simulink model "az_INDI_controller"  (R2023b)
settings: Solver=FixedStepAuto  StartTime=0.0  StopTime=8  FixedStep=0.001  RelTol=1e-3  AbsTol=1e-6
PreLoadFcn:
  | %aero_guid_dat
StopFcn:
  | %aero_guid_plot
undefined symbols (not defined in the file or in its folder): alpha_vec, Cm_alpha, Cm_el, Cm_q, Cx_alpha, Cz_alpha, Cz_el, d_ref, fin_max, fin_maxrate, fin_min, g, h_ini, Iyy, l_acc, Mach_vec, mass, q_ini, S_ref, Thrust, v_ini, x_ini
libraries: aerolibasang x3, aerolibatmos2 x1, aerolibactuator x1, simulink x1
CloseFcn:
  | h=findobj('type','figure');if ~isempty(h);close(h);end
Description:
  | Dynamics of a missile engaging a target which is flying straight and level
settings Model: Creator=The MathWorks, Inc.  LastModifiedBy=luzhi
settings SolverCC: AutoScaleAbsTol=off  AlgebraicLoopSolver=TrustRegion
settings DataIOCC: SaveFormat=Array  SaveOutput=off  ReturnWorkspaceOutputs=off  StateSaveName=xbase  OutputSaveName=ybase  SignalLoggingName=sigsOut
settings OptimizationCC: BlockReduction=off  ReuseModelBlockBuffer=off  ExpressionDepthLimit=2147483647  InitFltsAndDblsToZero=on  LifeSpan=inf
settings DebuggingCC: SaveWithParameterizedLinksMsg=none  SignalResolutionControl=TryResolveAllWithWarning  MultiTaskDSMMsg=warning  MultiTaskCondExecSysMsg=none  SigSpecEnsureSampleTimeMsg=none  FcnCallInpInsideContextMsg=warning  UnconnectedInputMsg=warning  UnconnectedOutputMsg=warning  UnconnectedLineMsg=warning  StateNameClashWarn=warning  SFUnexpectedBacktrackingDiag=warning  SFNoUnconditionalDefaultTransitionDiag=warning  SFExecutionAtInitializationDiag=none  ArithmeticOperatorsInVariantConditions=warning
settings HardwareCC: ProdBitPerPointer=32  ProdBitPerSizeT=32  ProdBitPerPtrDiffT=32  ProdLargestAtomicFloat=None  ProdIntDivRoundTo=Undefined  ProdEndianess=Unspecified  ProdWordSize=32  ProdHWDeviceType=32-bit Generic
settings ModelReferenceCC: EnableRefExpFcnMdlSchedulingChecks=on  PropagateSignalLabelsOutOfModel=off
settings SFSimCC: SimUseLocalCustomCode=off  SimParseCustomCode=off  CustomCodeUndefinedFunction=UseInterfaceOnly
settings RTWCC: RTWUseLocalCustomCode=off
settings CodeAppCC: StateflowObjectComments=on
settings GRTTargetCC: TargetFcnLib=ansi_tfl_tmw.mat  TargetLangStandard=C89/C90 (ANSI)  CombineOutputUpdateFcns=off  GRTInterface=on
settings ConfigComp: CovMetricSettings=d  CovSaveCumulativeToWorkspaceVar=on  CovSaveSingleToWorkspaceVar=on  CovExternalEMLEnable=off  CovSFcnEnable=off

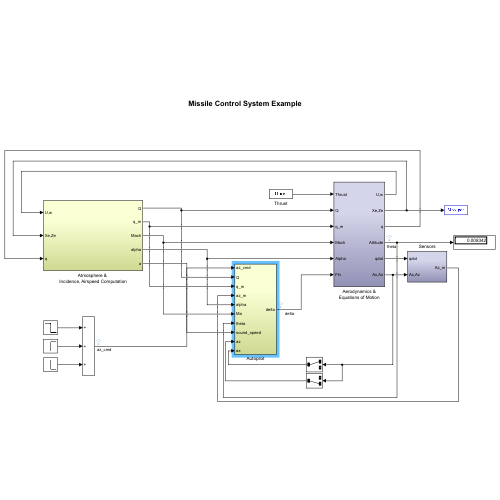
[thumbnail: Simulink's stored preview of the top-level diagram]
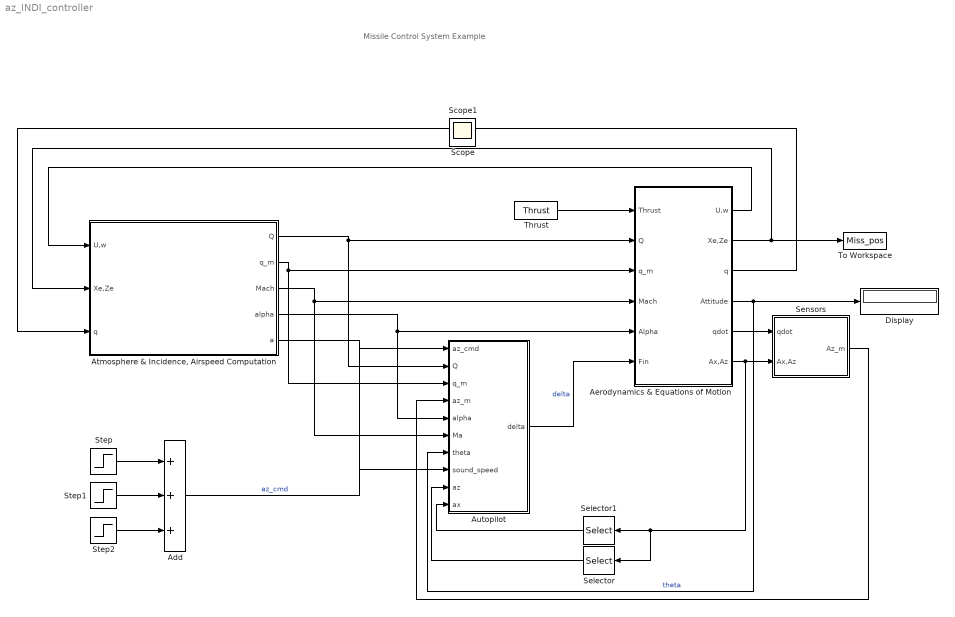
== system az_INDI_controller ==
  note: Missile Control System Example
  Add : Sum  Inputs=3
  Aerodynamics & Equations of Motion : Subsystem
  "Atmosphere & Incidence, Airspeed Computation" : Subsystem
  Autopilot : Subsystem
  Display : Display
  Selector : Selector  InputPortWidth=2  IndexOptions=Index vector (dialog)  Indices=[2]  OutputSizes=1
  Selector1 : Selector  InputPortWidth=2  IndexOptions=Index vector (dialog)  Indices=1  OutputSizes=1
  Sensors : Subsystem
  Step : Step  After=-10  SampleTime=0
  Step1 : Step  Time=3  After=20  SampleTime=0
  Step2 : Step  Time=5  After=-10  SampleTime=0
  Thrust : Constant  Value=Thrust
  To Workspace : ToWorkspace  VariableName=Miss_pos  SaveFormat=Structure With Time  SampleTime=-1
  Scope : Scope
  Scope1 : Scope
  wires:
  Autopilot/1(delta) -> Aerodynamics & Equations of Motion/6(Fin)  "delta"
  Aerodynamics & Equations of Motion/6(Ax,Az) -> Selector1/1, Selector/1, Sensors/2(Ax,Az)
  Aerodynamics & Equations of Motion/5(qdot) -> Sensors/1(qdot)
  Aerodynamics & Equations of Motion/4(Attitude) -> Autopilot/7(theta), Display/1  "theta"
  "Atmosphere & Incidence, Airspeed Computation"/2(q_m) -> Aerodynamics & Equations of Motion/3(q_m), Autopilot/3(q_m)
  "Atmosphere & Incidence, Airspeed Computation"/4(alpha) -> Autopilot/5(alpha), Aerodynamics & Equations of Motion/5(Alpha)
  "Atmosphere & Incidence, Airspeed Computation"/1(Q) -> Autopilot/2(Q), Aerodynamics & Equations of Motion/2(Q)
  Aerodynamics & Equations of Motion/1(U,w) -> "Atmosphere & Incidence, Airspeed Computation"/1(U,w)
  "Atmosphere & Incidence, Airspeed Computation"/3(Mach) -> Autopilot/6(Ma), Aerodynamics & Equations of Motion/4(Mach)
  Aerodynamics & Equations of Motion/2(Xe,Ze) -> To Workspace/1, "Atmosphere & Incidence, Airspeed Computation"/2(Xe,Ze)
  Aerodynamics & Equations of Motion/3(q) -> "Atmosphere & Incidence, Airspeed Computation"/3(q)
  Thrust/1 -> Aerodynamics & Equations of Motion/1(Thrust)
  Sensors/1(Az_m) -> Autopilot/4(az_m)
  "Atmosphere & Incidence, Airspeed Computation"/5(a) -> Autopilot/8(sound_speed)
  Selector/1 -> Autopilot/9(az)
  Add/1 -> Autopilot/1(az_cmd)  "az_cmd"
  Step/1 -> Add/1
  Step1/1 -> Add/2
  Step2/1 -> Add/3
  Selector1/1 -> Autopilot/10(ax)

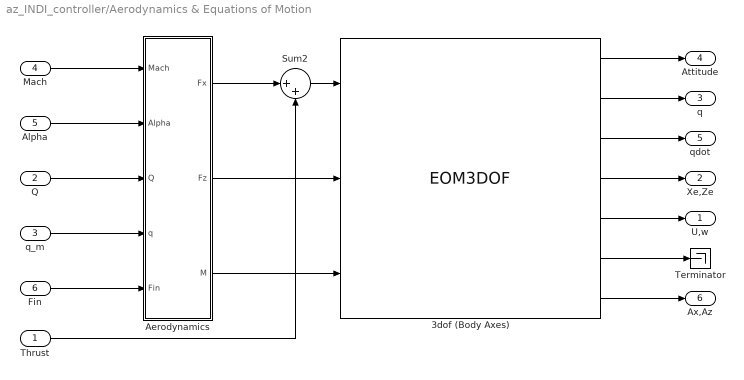
== system az_INDI_controller/Aerodynamics & Equations of Motion ==
  Thrust : Inport
  Q : Inport  Port=2
  q_m : Inport  Port=3
  Mach : Inport  Port=4
  Alpha : Inport  Port=5
  Fin : Inport  Port=6
  3dof (Body Axes) : EOM3DOF  v_ini=v_ini  theta_ini=theta_ini  q_ini=q_ini  alpha_ini=alpha_ini  pos_ini=[x_ini -h_ini]  mass=mass  Iyy=Iyy  g=g  abi_flag=on
  Aerodynamics : Subsystem
  Sum2 : Sum  Inputs=|++  InputSameDT=on  SaturateOnIntegerOverflow=on  OutDataTypeStr=Inherit: Same as first input
  Terminator : Terminator
  U,w : Outport  InitialOutput=0  VectorParamsAs1DForOutWhenUnconnected=off
  Xe,Ze : Outport  Port=2  InitialOutput=0  VectorParamsAs1DForOutWhenUnconnected=off
  q : Outport  Port=3  InitialOutput=0  VectorParamsAs1DForOutWhenUnconnected=off
  Attitude : Outport  Port=4  InitialOutput=0  VectorParamsAs1DForOutWhenUnconnected=off
  qdot : Outport  Port=5  InitialOutput=0  VectorParamsAs1DForOutWhenUnconnected=off
  Ax,Az : Outport  Port=6  InitialOutput=0  VectorParamsAs1DForOutWhenUnconnected=off
  wires:
  Aerodynamics/3(" M") -> 3dof (Body Axes)/3
  Sum2/1 -> 3dof (Body Axes)/1
  Fin/1 -> Aerodynamics/5(Fin)
  Aerodynamics/2(Fz) -> 3dof (Body Axes)/2
  Aerodynamics/1(Fx) -> Sum2/1
  Thrust/1 -> Sum2/2
  q_m/1 -> Aerodynamics/4(q)
  Mach/1 -> Aerodynamics/1(Mach)
  Q/1 -> Aerodynamics/3(Q)
  Alpha/1 -> Aerodynamics/2(Alpha)
  3dof (Body Axes)/7 -> Ax,Az/1
  3dof (Body Axes)/6 -> Terminator/1
  3dof (Body Axes)/5 -> U,w/1
  3dof (Body Axes)/4 -> Xe,Ze/1
  3dof (Body Axes)/3 -> qdot/1
  3dof (Body Axes)/2 -> q/1
  3dof (Body Axes)/1 -> Attitude/1

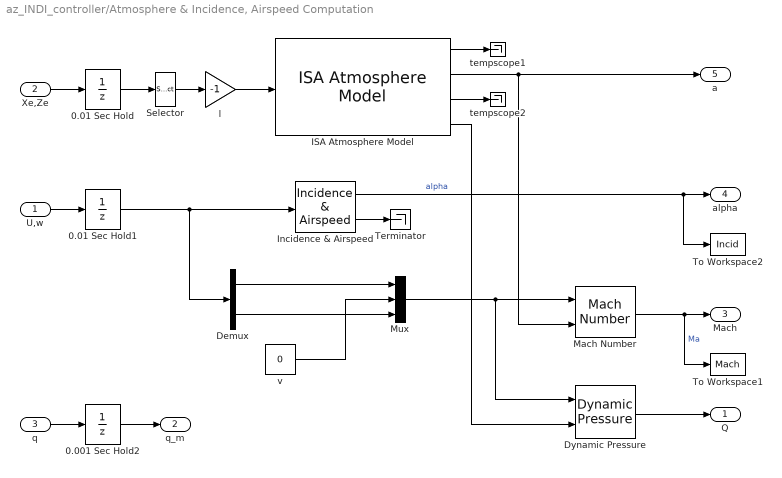
== system az_INDI_controller/Atmosphere & Incidence, Airspeed Computation ==
  U,w : Inport
  Xe,Ze : Inport  Port=2
  q : Inport  Port=3
  0.001 Sec Hold2 : UnitDelay  InitialCondition=q_ini  SampleTime=0.001  HasFrameUpgradeWarning=on
  0.01 Sec Hold : UnitDelay  InitialCondition=[x_ini -h_ini]  SampleTime=0.01  HasFrameUpgradeWarning=on
  0.01 Sec Hold1 : UnitDelay  InitialCondition=[v_ini 0]  SampleTime=0.01  HasFrameUpgradeWarning=on
  Demux : Demux  Outputs=2
  Dynamic Pressure : aerolibasang/Dynamic Pressure
  ISA Atmosphere Model : aerolibatmos2/ISA Atmosphere Model  useExtended=off  action=Warning  custom=off  viscosityOut=off  g=9.80665  gamma=1.4  R=287.0531  L=0.0065  h_trop=11000  h_strat=20000  rho0=1.225  P0=101325  T0=288.15  h0=0
  Incidence & Airspeed : aerolibasang/Incidence  & Airspeed
  Mach Number : aerolibasang/Mach Number
  Mux : Mux  Inputs=3
  Selector : Selector  InputPortWidth=2  IndexOptions=Index vector (dialog)  Indices=[2]  OutputSizes=1
  Terminator : Terminator
  To Workspace1 : ToWorkspace  VariableName=Mach  SaveFormat=Structure With Time  SampleTime=-1
  To Workspace2 : ToWorkspace  VariableName=Incid  SaveFormat=Structure With Time  SampleTime=-1
  l : Gain  Gain=-1  SaturateOnIntegerOverflow=on  OutDataTypeStr=Inherit: Same as input  ParamDataTypeStr=Inherit: Same as input
  tempscope1 : Terminator
  tempscope2 : Terminator
  v : Constant  Value=0
  Q : Outport
  q_m : Outport  Port=2
  Mach : Outport  Port=3
  alpha : Outport  Port=4
  a : Outport  Port=5
  wires:
  U,w/1 -> 0.01 Sec Hold1/1
  Incidence & Airspeed/1 -> To Workspace2/1, alpha/1  "alpha"
  Demux/1 -> Mux/1
  Demux/2 -> Mux/3
  v/1 -> Mux/2
  Mux/1 -> Mach Number/1, Dynamic Pressure/1
  Incidence & Airspeed/2 -> Terminator/1
  ISA Atmosphere Model/4 -> Dynamic Pressure/2
  Mach Number/1 -> To Workspace1/1, Mach/1  "Ma"
  Dynamic Pressure/1 -> Q/1
  0.01 Sec Hold1/1 -> Incidence & Airspeed/1, Demux/1
  0.01 Sec Hold/1 -> Selector/1
  l/1 -> ISA Atmosphere Model/1
  ISA Atmosphere Model/1 -> tempscope1/1
  ISA Atmosphere Model/3 -> tempscope2/1
  Selector/1 -> l/1
  Xe,Ze/1 -> 0.01 Sec Hold/1
  ISA Atmosphere Model/2 -> a/1, Mach Number/2
  0.001 Sec Hold2/1 -> q_m/1
  q/1 -> 0.001 Sec Hold2/1

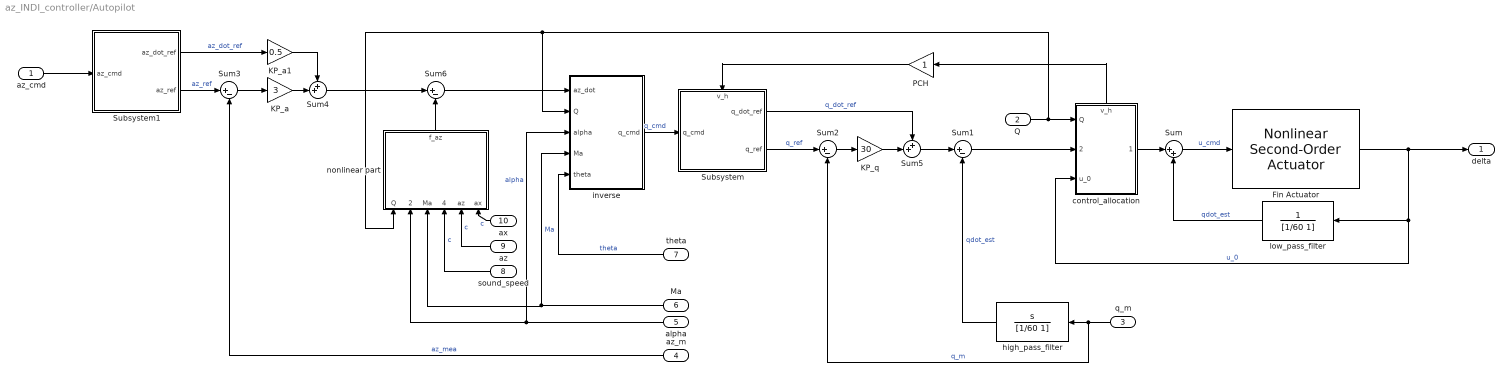
== system az_INDI_controller/Autopilot ==
  az_cmd : Inport
  Q : Inport  Port=2
  q_m : Inport  Port=3
  az_m : Inport  Port=4
  alpha : Inport  Port=5
  Ma : Inport  Port=6
  theta : Inport  Port=7
  sound_speed : Inport  Port=8
  az : Inport  Port=9
  ax : Inport  Port=10
  Fin Actuator : aerolibactuator/Nonlinear Second-Order Actuator  wn_fin=wn_fin  z_fin=z_fin  fin_max=fin_max  fin_min=fin_min  fin_maxrate=fin_maxrate  fin_act_0=fin_act_0  fin_act_vel=0
  KP_a : Gain  Gain=3
  KP_a1 : Gain  Gain=0.5
  KP_q : Gain  Gain=30
  PCH : Gain
  Subsystem : Subsystem
      settings: PortSchema="{\"entries\":[{\"content\":{\"sides\":[{\"content\":{\"connectorIds\":[\"In1\"]},\"type\":\"ConnectorPlacement.EquallySpacedRectSide\",\"uuid\":\"21326aec-3e5e-4acc-8d4b-147fb67c37ef\"},{\"content\":{\"connectorIds\":[\"Out1\",\"Out2\"],\"side\":\"RIGHT\"},\"type\":\"ConnectorPlacement.EquallySpacedRectSide\",\"uuid\":\"9c9abec6-e162-41f3-9a87-a5e646e431f6\"},{\"content\":{\"connectorIds\":[\"In2\"],\"side\":\"TOP\"},\"type\":\"ConnectorPlacement.EquallySpacedRectSide\",\"uuid\":\"37a4f4dd-e2ce-4d3c-ba5c-0e6f54d2f89b\"}]},\"type\":\"ConnectorPlacement.EquallySpacedConnector\",\"uuid\":\"006ee997-d3e3-4e6d-9e3d-0018891eb923\"}],\"packageUris\":[\"http://schema.mathworks.com/mf0/Connector/R2020b\"],\"version\":\"1.0\"}"
  Subsystem1 : Subsystem
  Sum : Sum  Inputs=|++
  Sum{1..3,6} (4 alike) : Sum  Inputs=|+-
  Sum4 : Sum  Inputs=++|
  Sum5 : Sum  Inputs=++|
  control_allocation : Subsystem
      settings: PortSchema="{\"entries\":[{\"content\":{\"sides\":[{\"content\":{\"connectorIds\":[\"In1\",\"In2\",\"In3\"]},\"type\":\"ConnectorPlacement.EquallySpacedRectSide\",\"uuid\":\"a0ce9da5-1ffc-4f75-9763-d32b58958b30\"},{\"content\":{\"connectorIds\":[\"Out1\"],\"side\":\"RIGHT\"},\"type\":\"ConnectorPlacement.EquallySpacedRectSide\",\"uuid\":\"34e52099-0fbe-4ef7-a509-693d90ad8665\"},{\"content\":{\"connectorIds\":[\"Out2\"],\"side\":\"TOP\"},\"type\":\"ConnectorPlacement.EquallySpacedRectSide\",\"uuid\":\"02b44c40-6b1e-4ed6-9dfc-88d3b20cdc66\"}]},\"type\":\"ConnectorPlacement.EquallySpacedConnector\",\"uuid\":\"9b53b305-2d8c-4631-9888-cc5118213f1a\"}],\"packageUris\":[\"http://schema.mathworks.com/mf0/Connector/R2020b\"],\"version\":\"1.0\"}"
  high_pass_filter : TransferFcn  Numerator=[1 0]  Denominator=[1/60 1]
  inverse : Subsystem
  low_pass_filter : TransferFcn  Denominator=[1/60 1]
  nonlinear part : Subsystem
  delta : Outport
  wires:
  Sum/1 -> Fin Actuator/1  "u_cmd"
  Fin Actuator/1 -> low_pass_filter/1, control_allocation/3(u_0), delta/1  "u_0"
  Q/1 -> inverse/2(Q), nonlinear part/1(Q), control_allocation/1(Q)
  Sum1/1 -> control_allocation/2(d_qdot)
  control_allocation/1(du_cmd) -> Sum/1
  high_pass_filter/1 -> Sum1/2  "qdot_est"
  q_m/1 -> Sum2/2, high_pass_filter/1  "q_m"
  low_pass_filter/1 -> Sum/2  "qdot_est"
  Sum2/1 -> KP_q/1
  KP_q/1 -> Sum5/2
  Sum5/1 -> Sum1/1
  Subsystem/1(q_dot_ref) -> Sum5/1  "q_dot_ref"
  Subsystem/2(q_ref) -> Sum2/1  "q_ref"
  control_allocation/2(v_h) -> PCH/1
  PCH/1 -> Subsystem/2(v_h)
  Subsystem1/2(az_ref) -> Sum3/1  "az_ref"
  Sum3/1 -> KP_a/1
  az_m/1 -> Sum3/2  "az_mea"
  KP_a/1 -> Sum4/2
  Subsystem1/1(az_dot_ref) -> KP_a1/1  "az_dot_ref"
  Sum4/1 -> Sum6/1
  Sum6/1 -> inverse/1(az_dot)
  inverse/1(q_cmd) -> Subsystem/1(q_cmd)  "q_cmd"
  alpha/1 -> nonlinear part/2(alpha), inverse/3(alpha)  "alpha"
  Ma/1 -> inverse/4(Ma), nonlinear part/3(Ma)  "Ma"
  theta/1 -> inverse/5(theta)  "theta"
  nonlinear part/1(f_az) -> Sum6/2
  sound_speed/1 -> nonlinear part/4(sound_speed)  "c"
  az/1 -> nonlinear part/5(az)  "c"
  ax/1 -> nonlinear part/6(ax)  "c"
  KP_a1/1 -> Sum4/1
  az_cmd/1 -> Subsystem1/1(az_cmd)

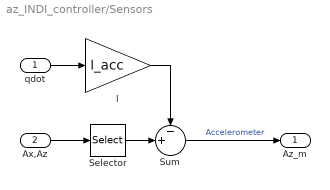
== system az_INDI_controller/Sensors ==
  qdot : Inport
  Ax,Az : Inport  Port=2
  Selector : Selector  InputPortWidth=2  IndexOptions=Index vector (dialog)  Indices=[2]  OutputSizes=1
  Sum : Sum  Inputs=-+|  InputSameDT=on  SaturateOnIntegerOverflow=on  OutDataTypeStr=Inherit: Same as first input
  l : Gain  Gain=l_acc  SaturateOnIntegerOverflow=on  OutDataTypeStr=Inherit: Same as input  ParamDataTypeStr=Inherit: Same as input
  Az_m : Outport  InitialOutput=0  VectorParamsAs1DForOutWhenUnconnected=off
  wires:
  Selector/1 -> Sum/2
  Ax,Az/1 -> Selector/1
  l/1 -> Sum/1
  Sum/1 -> Az_m/1  "Accelerometer"
  qdot/1 -> l/1

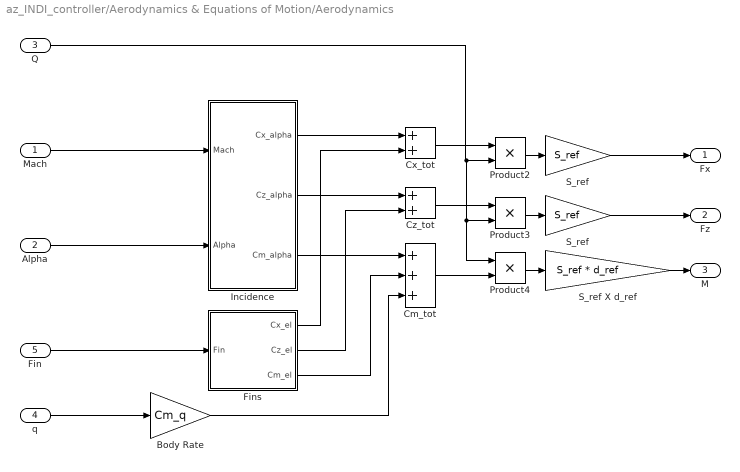
== system az_INDI_controller/Aerodynamics & Equations of Motion/Aerodynamics ==
  Mach : Inport
  Alpha : Inport  Port=2
  Q : Inport  Port=3
  q : Inport  Port=4
  Fin : Inport  Port=5
  Body Rate : Gain  Gain=Cm_q  SaturateOnIntegerOverflow=on  OutDataTypeStr=Inherit: Same as input  ParamDataTypeStr=Inherit: Same as input
  Cm_tot : Sum  Inputs=+++  InputSameDT=on  SaturateOnIntegerOverflow=on  OutDataTypeStr=Inherit: Same as first input
  Cx_tot : Sum  InputSameDT=on  SaturateOnIntegerOverflow=on  OutDataTypeStr=Inherit: Same as first input
  Cz_tot : Sum  InputSameDT=on  SaturateOnIntegerOverflow=on  OutDataTypeStr=Inherit: Same as first input
  Fins : Subsystem
  Incidence : Subsystem
  Product2 : Product  InputSameDT=on  SaturateOnIntegerOverflow=on  OutDataTypeStr=Inherit: Same as first input
  Product3 : Product  InputSameDT=on  SaturateOnIntegerOverflow=on  OutDataTypeStr=Inherit: Same as first input
  Product4 : Product  InputSameDT=on  SaturateOnIntegerOverflow=on  OutDataTypeStr=Inherit: Same as first input
  S_ref : Gain  Gain=S_ref  SaturateOnIntegerOverflow=on  OutDataTypeStr=Inherit: Same as input  ParamDataTypeStr=Inherit: Same as input
  "S_ref " : Gain  Gain=S_ref  SaturateOnIntegerOverflow=on  OutDataTypeStr=Inherit: Same as input  ParamDataTypeStr=Inherit: Same as input
  S_ref X d_ref : Gain  Gain=S_ref * d_ref  SaturateOnIntegerOverflow=on  OutDataTypeStr=Inherit: Same as input  ParamDataTypeStr=Inherit: Same as input
  Fx : Outport  InitialOutput=[0]  VectorParamsAs1DForOutWhenUnconnected=off
  Fz : Outport  Port=2  InitialOutput=0  VectorParamsAs1DForOutWhenUnconnected=off
  " M" : Outport  Port=3  InitialOutput=0  VectorParamsAs1DForOutWhenUnconnected=off
  wires:
  Incidence/1(Cx_alpha) -> Cx_tot/1
  Fins/1(Cx_el) -> Cx_tot/2
  Incidence/2(Cz_alpha) -> Cz_tot/1
  Fins/2(Cz_el) -> Cz_tot/2
  Incidence/3(Cm_alpha) -> Cm_tot/1
  Fins/3(Cm_el) -> Cm_tot/2
  Body Rate/1 -> Cm_tot/3
  Alpha/1 -> Incidence/2(Alpha)
  Cx_tot/1 -> Product2/1
  Cz_tot/1 -> Product3/1
  Product2/1 -> S_ref/1
  S_ref/1 -> Fx/1
  Product3/1 -> "S_ref "/1
  "S_ref "/1 -> Fz/1
  Fin/1 -> Fins/1(Fin)
  S_ref X d_ref/1 -> " M"/1
  Product4/1 -> S_ref X d_ref/1
  Cm_tot/1 -> Product4/2
  Mach/1 -> Incidence/1(Mach)
  q/1 -> Body Rate/1
  Q/1 -> Product4/1, Product3/2, Product2/2

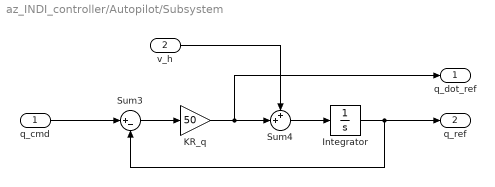
== system az_INDI_controller/Autopilot/Subsystem ==
  q_cmd : Inport
  v_h : Inport  Port=2
  Integrator : Integrator  LimitOutput=on  UpperSaturationLimit=pi/2  LowerSaturationLimit=-pi/2
  KR_q : Gain  Gain=50
  Sum3 : Sum  Inputs=|+-
  Sum4 : Sum  Inputs=++|
  q_dot_ref : Outport
  q_ref : Outport  Port=2
  wires:
  Sum4/1 -> Integrator/1
  v_h/1 -> Sum4/1
  KR_q/1 -> q_dot_ref/1, Sum4/2
  Integrator/1 -> q_ref/1, Sum3/2
  q_cmd/1 -> Sum3/1
  Sum3/1 -> KR_q/1

== system az_INDI_controller/Autopilot/Subsystem1 ==
  az_cmd : Inport
  Integrator : Integrator  LimitOutput=on  UpperSaturationLimit=30  LowerSaturationLimit=-30
  KR_az : Gain  Gain=10
  Sum3 : Sum  Inputs=|+-
  az_dot_ref : Outport
  az_ref : Outport  Port=2
  wires:
  KR_az/1 -> Integrator/1, az_dot_ref/1
  Integrator/1 -> az_ref/1, Sum3/2
  az_cmd/1 -> Sum3/1
  Sum3/1 -> KR_az/1

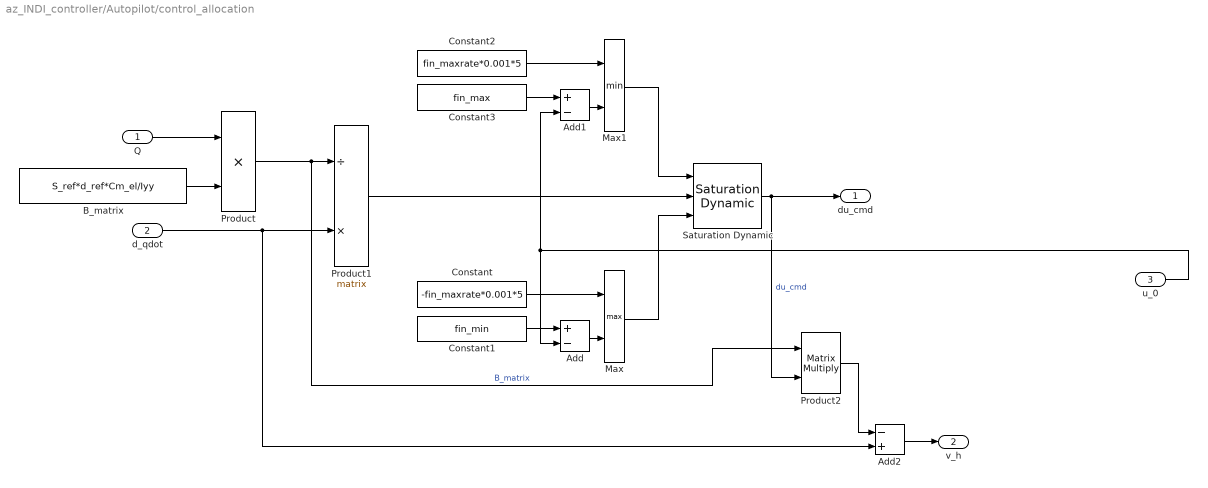
== system az_INDI_controller/Autopilot/control_allocation ==
  Q : Inport
  d_qdot : Inport  Port=2
  u_0 : Inport  Port=3
  Add : Sum  Inputs=+-
  Add1 : Sum  Inputs=+-
  Add2 : Sum  Inputs=-+
  B_matrix : Constant  Value=S_ref*d_ref*Cm_el/Iyy  VectorParams1D=off
  Constant : Constant  Value=-fin_maxrate*0.001*5  VectorParams1D=off
  Constant1 : Constant  Value=fin_min  VectorParams1D=off
  Constant2 : Constant  Value=fin_maxrate*0.001*5  VectorParams1D=off
  Constant3 : Constant  Value=fin_max  VectorParams1D=off
  Max : MinMax  Function=max  Inputs=2
  Max1 : MinMax  Inputs=2
  Product : Product
  Product1 : Product  Inputs=/*  Multiplication=Matrix(*)
  Product2 : Product  Multiplication=Matrix(*)
  Saturation Dynamic : simulink/Discontinuities/Saturation Dynamic  OutMin=[]  OutMax=[]  OutDataTypeStr=Inherit: Same as second input  OutDataType=fixdt(1, 16)  OutScaling=2^-10  DoSatur=off
  du_cmd : Outport
  v_h : Outport  Port=2
  wires:
  Add/1 -> Max/2
  B_matrix/1 -> Product/2
  d_qdot/1 -> Add2/2, Product1/2
  Constant2/1 -> Max1/1
  u_0/1 -> Add/2, Add1/2
  Constant/1 -> Max/1
  Add1/1 -> Max1/2
  Product/1 -> Product2/1, Product1/1  "B_matrix"
  Max/1 -> Saturation Dynamic/3
  Constant1/1 -> Add/1
  Q/1 -> Product/1
  Product1/1 -> Saturation Dynamic/2
  Constant3/1 -> Add1/1
  Max1/1 -> Saturation Dynamic/1
  Saturation Dynamic/1 -> Product2/2, du_cmd/1  "du_cmd"
  Product2/1 -> Add2/1
  Add2/1 -> v_h/1

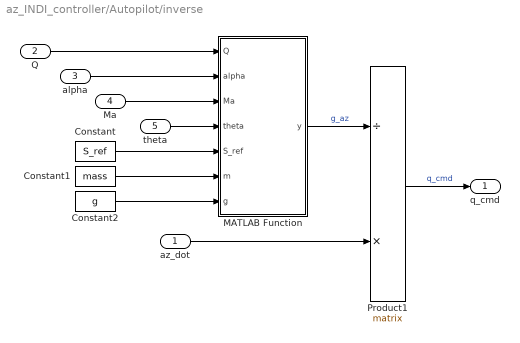
== system az_INDI_controller/Autopilot/inverse ==
  az_dot : Inport
  Q : Inport  Port=2
  alpha : Inport  Port=3
  Ma : Inport  Port=4
  theta : Inport  Port=5
  Constant : Constant  Value=S_ref
  Constant1 : Constant  Value=mass
  Constant2 : Constant  Value=g
  MATLAB Function : MATLAB Function  TreatAsAtomicUnit=on
  Product1 : Product  Inputs=/*  Multiplication=Matrix(*)
  q_cmd : Outport
  wires:
  Product1/1 -> q_cmd/1  "q_cmd"
  MATLAB Function/1(y) -> Product1/1  "g_az"
  az_dot/1 -> Product1/2
  Q/1 -> MATLAB Function/1(Q)
  alpha/1 -> MATLAB Function/2(alpha)
  Ma/1 -> MATLAB Function/3(Ma)
  theta/1 -> MATLAB Function/4(theta)
  Constant/1 -> MATLAB Function/5(S_ref)
  Constant1/1 -> MATLAB Function/6(m)
  Constant2/1 -> MATLAB Function/7(g)

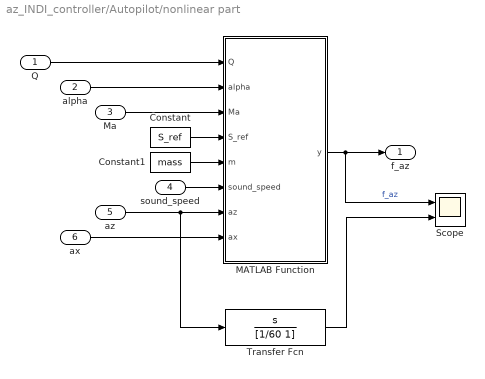
== system az_INDI_controller/Autopilot/nonlinear part ==
  Q : Inport
  alpha : Inport  Port=2
  Ma : Inport  Port=3
  sound_speed : Inport  Port=4
  az : Inport  Port=5
  ax : Inport  Port=6
  Constant : Constant  Value=S_ref
  Constant1 : Constant  Value=mass
  MATLAB Function : MATLAB Function  TreatAsAtomicUnit=on
  Scope : Scope  NumInputPorts=2
  Transfer Fcn : TransferFcn  Numerator=[1 0]  Denominator=[1/60 1]
  f_az : Outport
  wires:
  Q/1 -> MATLAB Function/1(Q)
  sound_speed/1 -> MATLAB Function/6(sound_speed)
  Ma/1 -> MATLAB Function/3(Ma)
  az/1 -> Transfer Fcn/1, MATLAB Function/7(az)
  alpha/1 -> MATLAB Function/2(alpha)
  Constant/1 -> MATLAB Function/4(S_ref)
  Constant1/1 -> MATLAB Function/5(m)
  ax/1 -> MATLAB Function/8(ax)
  Transfer Fcn/1 -> Scope/2
  MATLAB Function/1(y) -> f_az/1, Scope/1  "f_az"

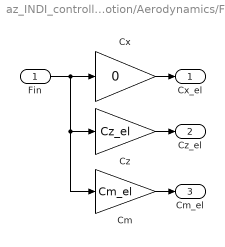
== system az_INDI_controller/Aerodynamics & Equations of Motion/Aerodynamics/Fins ==
  Fin : Inport
  Cm : Gain  Gain=Cm_el  SaturateOnIntegerOverflow=on  OutDataTypeStr=Inherit: Same as input  ParamDataTypeStr=Inherit: Same as input
  Cx : Gain  Gain=0  SaturateOnIntegerOverflow=on  OutDataTypeStr=Inherit: Same as input  ParamDataTypeStr=Inherit: Same as input
  Cz : Gain  Gain=Cz_el  SaturateOnIntegerOverflow=on  OutDataTypeStr=Inherit: Same as input  ParamDataTypeStr=Inherit: Same as input
  Cx_el : Outport  InitialOutput=0  VectorParamsAs1DForOutWhenUnconnected=off
  Cz_el : Outport  Port=2  InitialOutput=0  VectorParamsAs1DForOutWhenUnconnected=off
  Cm_el : Outport  Port=3  InitialOutput=0  VectorParamsAs1DForOutWhenUnconnected=off
  wires:
  Fin/1 -> Cx/1, Cm/1, Cz/1
  Cx/1 -> Cx_el/1
  Cm/1 -> Cm_el/1
  Cz/1 -> Cz_el/1

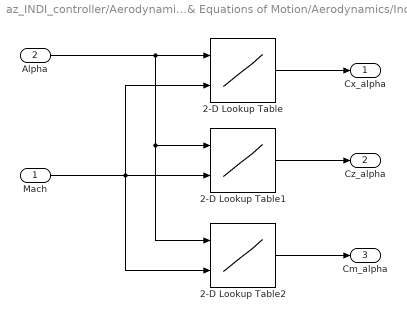
== system az_INDI_controller/Aerodynamics & Equations of Motion/Aerodynamics/Incidence ==
  Mach : Inport
  Alpha : Inport  Port=2
  2-D Lookup Table : Lookup_n-D  BreakpointsForDimension1=alpha_vec  BreakpointsForDimension2=Mach_vec  Table=Cx_alpha  InternalRulePriority=Speed  RndMeth=Simplest
      settings: InputPortMap=u0,u1
  2-D Lookup Table1 : Lookup_n-D  BreakpointsForDimension1=alpha_vec  BreakpointsForDimension2=Mach_vec  Table=Cz_alpha  InternalRulePriority=Speed  RndMeth=Simplest
      settings: InputPortMap=u0,u1
  2-D Lookup Table2 : Lookup_n-D  BreakpointsForDimension1=alpha_vec  BreakpointsForDimension2=Mach_vec  Table=Cm_alpha  InternalRulePriority=Speed  RndMeth=Simplest
      settings: InputPortMap=u0,u1
  Cx_alpha : Outport  InitialOutput=0  VectorParamsAs1DForOutWhenUnconnected=off
  Cz_alpha : Outport  Port=2  InitialOutput=0  VectorParamsAs1DForOutWhenUnconnected=off
  Cm_alpha : Outport  Port=3  InitialOutput=0  VectorParamsAs1DForOutWhenUnconnected=off
  wires:
  Alpha/1 -> 2-D Lookup Table/1, 2-D Lookup Table2/1, 2-D Lookup Table1/1
  2-D Lookup Table/1 -> Cx_alpha/1
  2-D Lookup Table1/1 -> Cz_alpha/1
  Mach/1 -> 2-D Lookup Table2/2, 2-D Lookup Table1/2, 2-D Lookup Table/2
  2-D Lookup Table2/1 -> Cm_alpha/1

== matlab function az_INDI_controller/Autopilot/nonlinear part/MATLAB Function ==
  data: Q input; y output; alpha input; Ma input; S_ref input; m input; sound_speed input; az input; ax input
function y = fcn(Q, alpha, Ma, S_ref, m, sound_speed, az, ax)

V = max(10, Ma * sound_speed);
dCz_dalpha = -19.5264 + 61.0047*abs(alpha) + 55.6785*alpha^2 + 3.2391*Ma;
y = Q*S_ref/m * dCz_dalpha * (az*cos(alpha) - ax*sin(alpha))/V;
end

== matlab function az_INDI_controller/Autopilot/inverse/MATLAB Function ==
  data: Q input; y output; alpha input; Ma input; theta input; S_ref input; m input; g input
function y = fcn(Q, alpha, Ma, theta, S_ref, m, g)

dCz_dalpha = -19.5264 + 61.0047*abs(alpha) + 55.6785*alpha^2 + 3.2391*Ma;
y = Q*S_ref/m * dCz_dalpha - g*sin(theta);
end
